simulink model "Jacobian_and_IJacobian_Func_Simulink"  (R2021a)
settings: Solver=VariableStepAuto  StartTime=0.0  StopTime=10.0  RelTol=1e-3
settings Model: Creator=WU  LastModifiedBy=WU

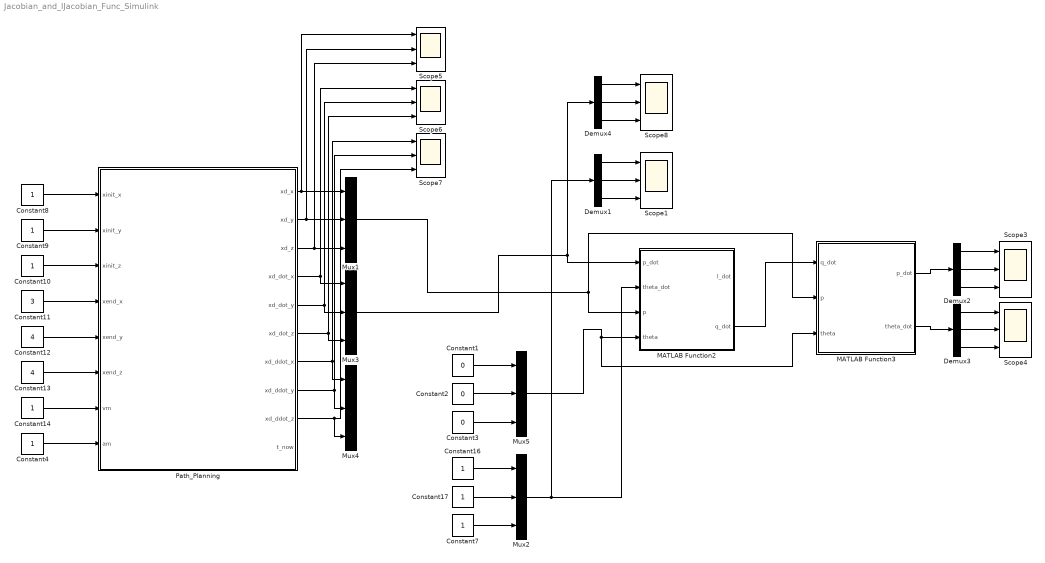
== system Jacobian_and_IJacobian_Func_Simulink ==
  Constant1 : Constant  Value=0  VectorParams1D=off
  Constant{4,7,9..10,14,17} (6 alike) : Constant
  Constant11 : Constant  Value=3
  Constant12 : Constant  Value=4
  Constant13 : Constant  Value=4
  Constant16 : Constant  VectorParams1D=off
  Constant2 : Constant  Value=0
  Constant3 : Constant  Value=0
  Constant8 : Constant  VectorParams1D=off
  Demux{1..4} (4 alike) : Demux  Outputs=3
      settings: DisplayOption=none
  MATLAB Function2 : MATLAB Function  TreatAsAtomicUnit=on
  MATLAB Function3 : MATLAB Function  TreatAsAtomicUnit=on
  Mux{1..5} (5 alike) : Mux  Inputs=3
  Path_Planning : Subsystem
  Scope{1,3..8} (7 alike) : Scope  NumInputPorts=3
  wires:
  MATLAB Function3/2(theta_dot) -> Demux3/1
  Demux3/3 -> Scope4/3
  Demux2/1 -> Scope3/1
  Demux2/3 -> Scope3/3
  Demux3/2 -> Scope4/2
  MATLAB Function3/1(p_dot) -> Demux2/1
  Demux4/2 -> Scope8/2
  Demux4/3 -> Scope8/3
  Demux4/1 -> Scope8/1
  Demux3/1 -> Scope4/1
  Demux2/2 -> Scope3/2
  MATLAB Function2/2(q_dot) -> MATLAB Function3/1(q_dot)
  Constant10/1 -> Path_Planning/3(xinit_z)
  Path_Planning/1(xd_x) -> Scope5/1, Mux1/1
  Path_Planning/2(xd_y) -> Scope5/2, Mux1/2
  Path_Planning/8(xd_ddot_y) -> Scope7/2, Mux4/2
  Path_Planning/7(xd_ddot_x) -> Scope7/1, Mux4/1
  Constant12/1 -> Path_Planning/5(xend_y)
  Constant14/1 -> Path_Planning/7(vm)
  Constant11/1 -> Path_Planning/4(xend_x)
  Path_Planning/6(xd_dot_z) -> Scope6/3, Mux3/3
  Constant9/1 -> Path_Planning/2(xinit_y)
  Constant8/1 -> Path_Planning/1(xinit_x)
  Path_Planning/3(xd_z) -> Scope5/3, Mux1/3
  Constant13/1 -> Path_Planning/6(xend_z)
  Path_Planning/4(xd_dot_x) -> Scope6/1, Mux3/1
  Path_Planning/9(xd_ddot_z) -> Scope7/3, Mux4/3
  Path_Planning/5(xd_dot_y) -> Scope6/2, Mux3/2
  Mux3/1 -> Demux4/1, MATLAB Function2/1(p_dot)
  Constant2/1 -> Mux5/2
  Constant7/1 -> Mux2/3
  Constant1/1 -> Mux5/1
  Constant16/1 -> Mux2/1
  Constant3/1 -> Mux5/3
  Constant17/1 -> Mux2/2
  Mux5/1 -> MATLAB Function3/3(theta), MATLAB Function2/4(theta)
  Mux2/1 -> Demux1/1, MATLAB Function2/2(theta_dot)
  Mux1/1 -> MATLAB Function3/2(p), MATLAB Function2/3(p)
  Demux1/3 -> Scope1/3
  Demux1/1 -> Scope1/1
  Demux1/2 -> Scope1/2
  Constant4/1 -> Path_Planning/8(am)

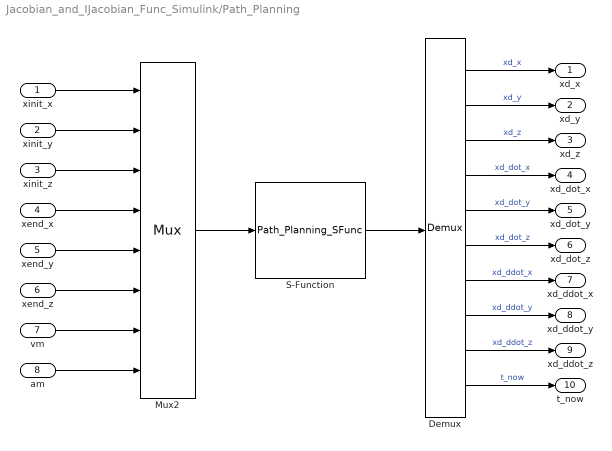
== system Jacobian_and_IJacobian_Func_Simulink/Path_Planning ==
  xinit_x : Inport
  xinit_y : Inport  Port=2
  xinit_z : Inport  Port=3
  xend_x : Inport  Port=4
  xend_y : Inport  Port=5
  xend_z : Inport  Port=6
  vm : Inport  Port=7
  am : Inport  Port=8
  Demux : Demux  Outputs=10
      settings: DisplayOption=none
  Mux2 : Mux  Inputs=8
  S-Function : S-Function  FunctionName=Path_Planning_SFunc  SFunctionDeploymentMode=off  EnableBusSupport=off
  xd_x : Outport
  xd_y : Outport  Port=2
  xd_z : Outport  Port=3
  xd_dot_x : Outport  Port=4
  xd_dot_y : Outport  Port=5
  xd_dot_z : Outport  Port=6
  xd_ddot_x : Outport  Port=7
  xd_ddot_y : Outport  Port=8
  xd_ddot_z : Outport  Port=9
  t_now : Outport  Port=10
  wires:
  Demux/7 -> xd_ddot_x/1  "xd_ddot_x"
  vm/1 -> Mux2/7
  xinit_y/1 -> Mux2/2
  Demux/1 -> xd_x/1  "xd_x"
  Demux/4 -> xd_dot_x/1  "xd_dot_x"
  Demux/5 -> xd_dot_y/1  "xd_dot_y"
  Demux/9 -> xd_ddot_z/1  "xd_ddot_z"
  Demux/8 -> xd_ddot_y/1  "xd_ddot_y"
  Demux/3 -> xd_z/1  "xd_z"
  Demux/6 -> xd_dot_z/1  "xd_dot_z"
  Demux/2 -> xd_y/1  "xd_y"
  xend_y/1 -> Mux2/5
  Mux2/1 -> S-Function/1
  S-Function/1 -> Demux/1
  xend_z/1 -> Mux2/6
  xend_x/1 -> Mux2/4
  xinit_z/1 -> Mux2/3
  xinit_x/1 -> Mux2/1
  am/1 -> Mux2/8
  Demux/10 -> t_now/1  "t_now"

== matlab function Jacobian_and_IJacobian_Func_Simulink/MATLAB Function2 ==
  data: p_dot input; theta_dot input; l_dot output; p input; theta input; q_dot output
function [l_dot,q_dot] = Jacobian_Func(p_dot,theta_dot,p,theta)
% 雅可比矩阵，从位姿x到绳长l，再到电机角度q

x=theta(1);
y=theta(2);
z=theta(3);
Rxyz=Theta2RotationMatrix_Func(x,y,z);

%% CoGiRo的参数 8绳索6自由度的CDPRs
% ai的定义
a1=[-7.5 -5.5 6]';
a2=[-7.5 -5.5 6]';
a3=[-7.5 5.5 6]';
a4=[-7.5 5.5 6]';
a5=[7.5 5.5 6]';
a6=[7.5 5.5 6]';
a7=[7.5 -5.5 6]';
a8=[7.5 -5.5 6]';
% bi的定义
b1=Rxyz*[0.5 -0.5 0]';
b2=Rxyz*[-0.5 0.5 1]';
b3=Rxyz*[-0.5 -0.5 0]';
b4=Rxyz*[0.5 0.5 1]';
b5=Rxyz*[-0.5 0.5 0]';
b6=Rxyz*[0.5 -0.5 1]';
b7=Rxyz*[0.5 0.5 0]';
b8=Rxyz*[-0.5 -0.5 1]';
% 绳索张力的上下限
tM=1000;
tm=10;
%% li=ai-bi-p,然后归一化li得到si=li/norm(li)
% li=ai-bi-p
l1=a1-b1-p;
l2=a2-b3-p;
l3=a3-b3-p;
l4=a4-b4-p;
l5=a5-b5-p;
l6=a6-b6-p;
l7=a7-b7-p;
l8=a8-b8-p;
% for i=1:8
%     expr=['l',num2str(i),'=a',num2str(i),'-b',num2str(i),'-p;'];
%     eval(expr);
% end
% si=li/norm(li)
s1=l1/norm(l1);
s2=l2/norm(l2);
s3=l3/norm(l3);
s4=l4/norm(l4);
s5=l5/norm(l5);
s6=l6/norm(l6);
s7=l7/norm(l7);
s8=l8/norm(l8);
% for i=1:8
%     expr=['s',num2str(i),'=l',num2str(i),'./norm(l',num2str(i),');'];
%     eval(expr);
% end

%% 构建W矩阵
% wi=[si;cross(bi,si)]
w1=[s1;cross(b1,s1)];
w2=[s2;cross(b2,s2)];
w3=[s3;cross(b3,s3)];
w4=[s4;cross(b4,s4)];
w5=[s5;cross(b5,s5)];
w6=[s6;cross(b6,s6)];
w7=[s7;cross(b7,s7)];
w8=[s8;cross(b8,s8)];
W=[w1 w2 w3 w4 w5 w6 w7 w8];

%% 得到雅可比矩阵
J=-W';

x_dot=[p_dot;theta_dot];

l_dot=J*x_dot;
q_dot=l_dot/0.0225;

end

== matlab function Jacobian_and_IJacobian_Func_Simulink/MATLAB Function3 ==
  data: q_dot input; p_dot output; p input; theta input; theta_dot output
function [p_dot,theta_dot] = Inverse_Jacobian_Func(q_dot,p,theta)
% 雅可比矩阵，从位姿x到绳长l，再到电机角度q

x=theta(1);
y=theta(2);
z=theta(3);
Rxyz=Theta2RotationMatrix_Func(x,y,z);

%% CoGiRo的参数 8绳索6自由度的CDPRs
% ai的定义
a1=[-7.5 -5.5 6]';
a2=[-7.5 -5.5 6]';
a3=[-7.5 5.5 6]';
a4=[-7.5 5.5 6]';
a5=[7.5 5.5 6]';
a6=[7.5 5.5 6]';
a7=[7.5 -5.5 6]';
a8=[7.5 -5.5 6]';
% bi的定义
b1=Rxyz*[0.5 -0.5 0]';
b2=Rxyz*[-0.5 0.5 1]';
b3=Rxyz*[-0.5 -0.5 0]';
b4=Rxyz*[0.5 0.5 1]';
b5=Rxyz*[-0.5 0.5 0]';
b6=Rxyz*[0.5 -0.5 1]';
b7=Rxyz*[0.5 0.5 0]';
b8=Rxyz*[-0.5 -0.5 1]';
% 绳索张力的上下限
tM=1000;
tm=10;
%% li=ai-bi-p,然后归一化li得到si=li/norm(li)
% li=ai-bi-p
l1=a1-b1-p;
l2=a2-b3-p;
l3=a3-b3-p;
l4=a4-b4-p;
l5=a5-b5-p;
l6=a6-b6-p;
l7=a7-b7-p;
l8=a8-b8-p;
% for i=1:8
%     expr=['l',num2str(i),'=a',num2str(i),'-b',num2str(i),'-p;'];
%     eval(expr);
% end
% si=li/norm(li)
s1=l1/norm(l1);
s2=l2/norm(l2);
s3=l3/norm(l3);
s4=l4/norm(l4);
s5=l5/norm(l5);
s6=l6/norm(l6);
s7=l7/norm(l7);
s8=l8/norm(l8);
% for i=1:8
%     expr=['s',num2str(i),'=l',num2str(i),'./norm(l',num2str(i),');'];
%     eval(expr);
% end

%% 构建W矩阵
% wi=[si;cross(bi,si)]
w1=[s1;cross(b1,s1)];
w2=[s2;cross(b2,s2)];
w3=[s3;cross(b3,s3)];
w4=[s4;cross(b4,s4)];
w5=[s5;cross(b5,s5)];
w6=[s6;cross(b6,s6)];
w7=[s7;cross(b7,s7)];
w8=[s8;cross(b8,s8)];
W=[w1 w2 w3 w4 w5 w6 w7 w8];

%% 得到雅可比矩阵
J=-W';
J_plus=pinv(J);
l_dot=q_dot*0.0225;
x_dot=J_plus*l_dot;
p_dot=x_dot(1:3,:);
theta_dot=x_dot(4:6,:);

end
